simulink model "CartPend"  (R2017a)
settings: Solver=ode45  StartTime=0.0  StopTime=1  RelTol=1e-3  EnableMultiTasking=on
values from neighbouring files (symbols this model uses):
  b = 0.1    [CartParams.m]
  g = 10    [CartParams.m]
  l = 0.3    [CartParams.m]
  m = 0.2    [CartParams.m]
  M = 0.5    [CartParams.m]
settings Model: Creator=Yanir  LastModifiedBy=hkariti
settings DataIOCC: LimitDataPoints=on  SaveFormat=Array
settings OptimizationCC: LifeSpan=inf
settings DebuggingCC: SFUnexpectedBacktrackingDiag=warning  SFNoUnconditionalDefaultTransitionDiag=warning  SFExecutionAtInitializationDiag=none
settings HardwareCC: ProdBitPerPointer=32  ProdBitPerSizeT=32  ProdBitPerPtrDiffT=32  ProdLargestAtomicFloat=None  ProdIntDivRoundTo=Undefined  ProdEndianess=Unspecified  ProdWordSize=32  ProdHWDeviceType=32-bit Generic
settings ModelReferenceCC: PropagateSignalLabelsOutOfModel=off
settings GRTTargetCC: TargetLangStandard=C89/C90 (ANSI)  GeneratePreprocessorConditionals=Disable all
settings ConfigComp: CovMetricSettings=dw  CovHtmlReporting=on  CovSaveCumulativeToWorkspaceVar=on  CovSaveSingleToWorkspaceVar=on  CovExternalEMLEnable=off

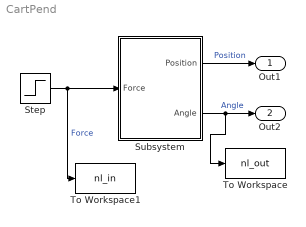
== system CartPend ==
  Step : Step  Time=0  SampleTime=0
  Subsystem : Subsystem
  To Workspace : ToWorkspace  VariableName=nl_out  SaveFormat=Timeseries  SampleTime=-1
  To Workspace1 : ToWorkspace  VariableName=nl_in  SaveFormat=Timeseries  SampleTime=-1
  Out1 : Outport
  Out2 : Outport  Port=2
  wires:
  Step/1 -> To Workspace1/1, Subsystem/1(Force)  "Force"
  Subsystem/1(Position) -> Out1/1  "Position"
  Subsystem/2(Angle) -> To Workspace/1, Out2/1  "Angle"

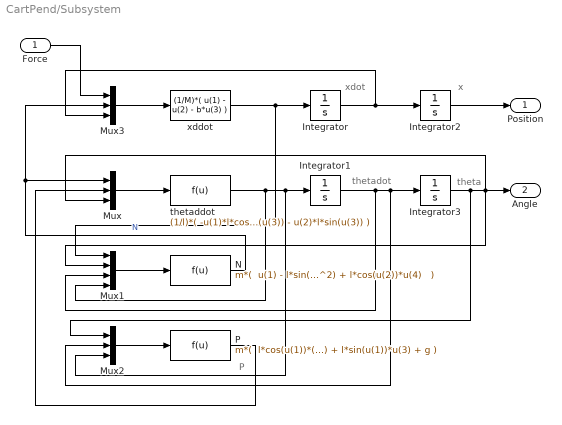
== system CartPend/Subsystem ==
  note: xdot
  note: x
  note: thetadot
  note: theta
  note: P
  Force : Inport
  Integrator : Integrator  ContinuousStateAttributes='xdot'
  Integrator1 : Integrator  ContinuousStateAttributes='thetadot'
  Integrator2 : Integrator  ContinuousStateAttributes='x'
  Integrator3 : Integrator  InitialCondition=pi  ContinuousStateAttributes='theta'
  Mux : Mux  Inputs=3
  Mux1 : Mux
  Mux2 : Mux  Inputs=3
  Mux3 : Mux  Inputs=3
  N : Fcn  Expr="m*(  u(1) - l*sin(u(2))*(u(3)^2) + l*cos(u(2))*u(4)   )"
  P : Fcn  Expr="m*(  l*cos(u(1))*(u(2)^2) + l*sin(u(1))*u(3) + g )"
  thetaddot : Fcn  Expr=(1/l)*( -u(1)*l*cos(u(3)) - u(2)*l*sin(u(3)) )
  xddot : Fcn  Expr=(1/M)*( u(1) - u(2) - b*u(3) )
  Position : Outport
  Angle : Outport  Port=2
  wires:
  Integrator/1 -> Integrator2/1, Mux3/3
  Integrator1/1 -> Mux1/3, Mux2/2, Integrator3/1
  xddot/1 -> Integrator/1, Mux1/1
  thetaddot/1 -> Mux1/4, Integrator1/1, Mux2/3
  Mux/1 -> thetaddot/1
  Integrator2/1 -> Position/1
  Integrator3/1 -> Mux1/2, Mux/3, Angle/1, Mux2/1
  Mux1/1 -> N/1
  Mux3/1 -> xddot/1
  Force/1 -> Mux3/1
  N/1 -> Mux3/2, Mux/1  "N"
  Mux2/1 -> P/1
  P/1 -> Mux/2
